simulink model "black_box_battery_2017compat"  (R2017b)
settings: Solver=FixedStepDiscrete  StartTime=0.0  StopTime=500  FixedStep=0.1  RelTol=1e-3
PreLoadFcn:
  | load('battery_final_portable_mux_demux_model.mat')
  | run('convert_c2d.m')
values from neighbouring files (symbols this model uses):
  A_d = [0.386994154142 0.130528867937 0.00753731445977 1.05252849992e-06 0 0 0 0 0 0 0 -0.260915565234 ... (121 elements, 11x11)]    [battery_final_discrete_for_simulink.mat]    (also in convert_c2d.m = battery_sys_d.A)
  B_d = [0.00407902712304 0.000471082153736 1.68404559988e-05 1.71473651939e-09 0 0 0 0 0 0 0 0 ... (44 elements, 11x4)]    [battery_final_discrete_for_simulink.mat]    (also in convert_c2d.m = battery_sys_d.B)
  C_d = [-0.0403469184323 0 0.00489964923997 0 -0.00193385654799 0 0.0091411610057 0 0.0963442624262 0 0.00960199809146 0 ... (22 elements, 2x11)]    [battery_final_discrete_for_simulink.mat]    (also in convert_c2d.m = battery_sys_d.C)
  D_d = [0  0  0  0; 0  0  0  0]    [battery_final_discrete_for_simulink.mat]    (also in convert_c2d.m = battery_sys_d.D)
  nx_final = 11    [battery_final_portable_mux_demux_model.mat]
undefined symbols (not defined in the file or in its folder): DiscIntNeverNeededParam
libraries: cstblocks x1, simulink x1
settings Model: Creator=ananthakrishnan.kaim  LastModifiedBy=ananthakrishnan.kaim

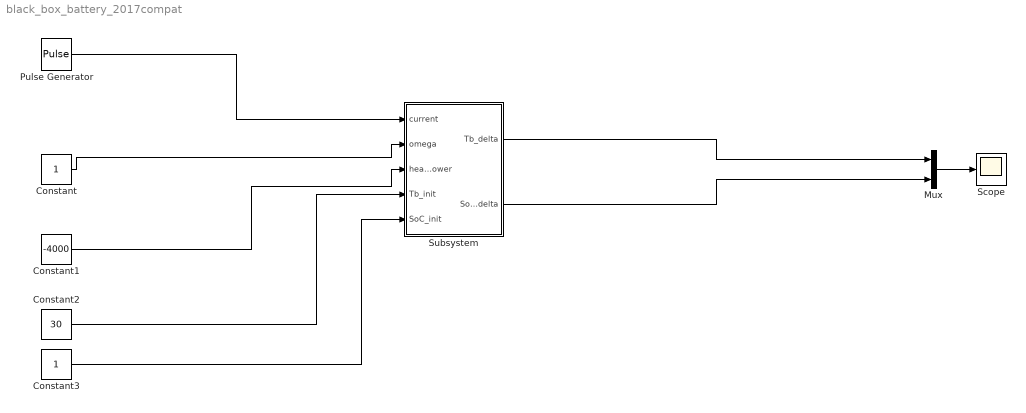
== system black_box_battery_2017compat ==
  Constant : Constant
  Constant1 : Constant  Value=-4000
  Constant2 : Constant  Value=30
  Constant3 : Constant
  Mux : Mux  Inputs=2
  Pulse Generator : DiscretePulseGenerator  PulseType=Time based  Amplitude=25  Period=100  PulseWidth=10
  Scope : Scope
  Subsystem : Subsystem
  wires:
  Pulse Generator/1 -> Subsystem/1(current)
  Constant/1 -> Subsystem/2(omega)
  Constant1/1 -> Subsystem/3(heat_power)
  Subsystem/1(Tb_delta) -> Mux/1
  Subsystem/2(SoC_delta) -> Mux/2
  Mux/1 -> Scope/1
  Constant2/1 -> Subsystem/4(Tb_init)
  Constant3/1 -> Subsystem/5(SoC_init)

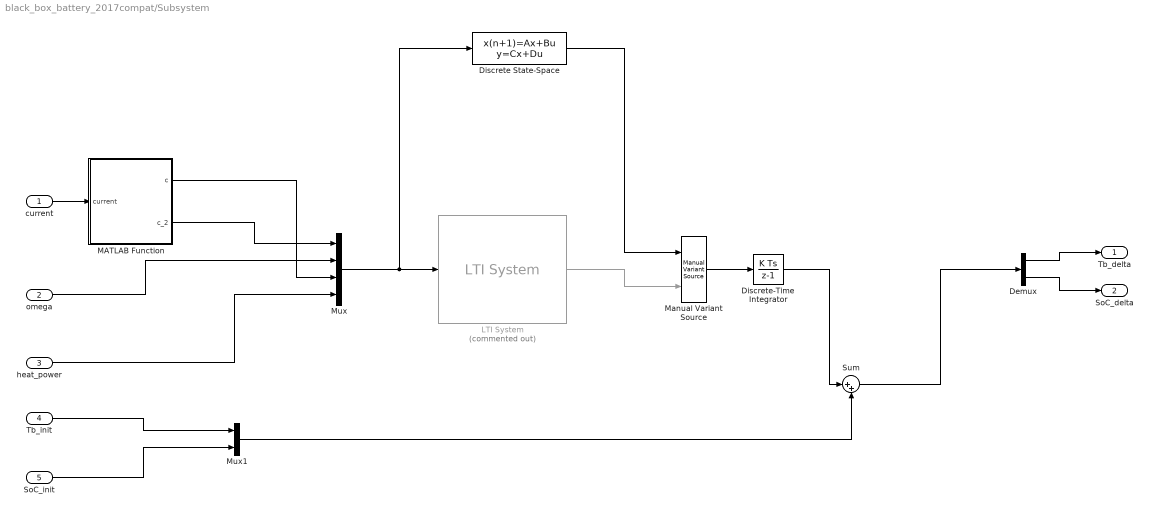
== system black_box_battery_2017compat/Subsystem ==
  current : Inport
  omega : Inport  Port=2
  heat_power : Inport  Port=3
  Tb_init : Inport  Port=4
  SoC_init : Inport  Port=5
  Demux : Demux  Outputs=2
  Discrete State-Space : DiscreteStateSpace  A=A_d  B=B_d  C=C_d  D=D_d  InitialCondition=zeros(nx_final,1)  SampleTime=-1
  Discrete-Time Integrator : DiscreteIntegrator  InitialConditionSetting=State (most efficient)  SampleTime=-1  ICPrevOutput=DiscIntNeverNeededParam  ICPrevScaledInput=DiscIntNeverNeededParam
  LTI System : cstblocks/LTI System  Commented=on  sys=TF_final  IC=[]
  MATLAB Function : MATLAB Function  TreatAsAtomicUnit=on
  Manual Variant Source : simulink/Signal Routing/Manual Variant Source  NumChoices=2  OverrideUsingVariant=V_1
      settings: SourceProductName=Simulink
  Mux : Mux
  Mux1 : Mux  Inputs=2
  Sum : Sum  Inputs=|++
  Tb_delta : Outport
  SoC_delta : Outport  Port=2
  wires:
  current/1 -> MATLAB Function/1(current)
  Mux/1 -> Discrete State-Space/1, LTI System/1
  MATLAB Function/1(c) -> Mux/3
  Demux/2 -> SoC_delta/1
  Demux/1 -> Tb_delta/1
  MATLAB Function/2(c_2) -> Mux/1
  Manual Variant Source/1 -> Discrete-Time Integrator/1
  heat_power/1 -> Mux/4
  omega/1 -> Mux/2
  Discrete State-Space/1 -> Manual Variant Source/1
  LTI System/1 -> Manual Variant Source/2
  Tb_init/1 -> Mux1/1
  SoC_init/1 -> Mux1/2
  Discrete-Time Integrator/1 -> Sum/1
  Mux1/1 -> Sum/2
  Sum/1 -> Demux/1

== matlab function black_box_battery_2017compat/Subsystem/MATLAB Function ==
  data: current input; c output; c_2 output
function [c,c_2] = fcn(current)
c_2=current^2;
c=current;
end
